simulink model "rightLegController"  (R2017b)
settings: Solver=VariableStepAuto  StartTime=0.0  StopTime=10.0  RelTol=1e-3
libraries: simulink x9, nesl_utility x9
settings Model: Creator=Kalana  LastModifiedBy=Kalana

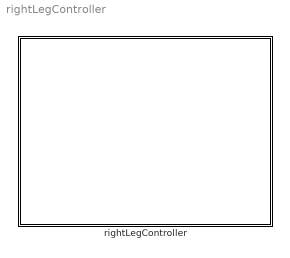
== system rightLegController ==
  "rightLegController " : Subsystem

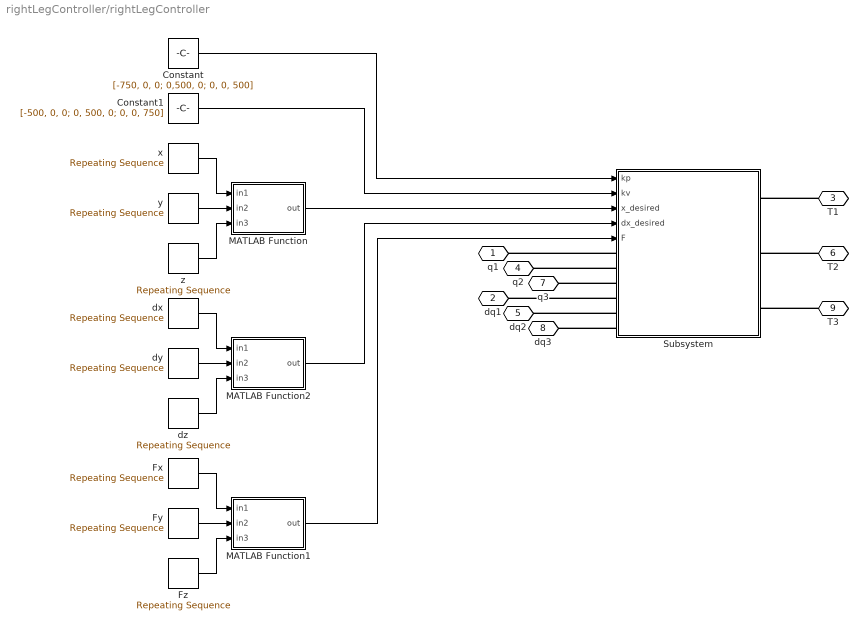
== system rightLegController/rightLegController  ==
  Constant : Constant  Value=[-750, 0, 0; 0,500, 0; 0, 0, 500]  VectorParams1D=off
  Constant1 : Constant  Value=[-500, 0, 0; 0, 500, 0; 0, 0, 750]  VectorParams1D=off
  Fx : simulink/Sources/Repeating Sequence  rep_seq_t=time_force  rep_seq_y=Fx
  Fy : simulink/Sources/Repeating Sequence  rep_seq_t=time_force  rep_seq_y=Fy
  Fz : simulink/Sources/Repeating Sequence  rep_seq_t=time_force  rep_seq_y=Fz
  MATLAB Function : MATLAB Function  TreatAsAtomicUnit=on
  MATLAB Function1 : MATLAB Function  TreatAsAtomicUnit=on
  MATLAB Function2 : MATLAB Function  TreatAsAtomicUnit=on
  Subsystem : Subsystem
  dx : simulink/Sources/Repeating Sequence  rep_seq_t=time_velo  rep_seq_y=Vx
  dy : simulink/Sources/Repeating Sequence  rep_seq_t=time_velo  rep_seq_y=Vy
  dz : simulink/Sources/Repeating Sequence  rep_seq_t=time_velo  rep_seq_y=Vz
  x : simulink/Sources/Repeating Sequence  rep_seq_t=time_pos  rep_seq_y=x
  y : simulink/Sources/Repeating Sequence  rep_seq_t=time_pos  rep_seq_y=y
  z : simulink/Sources/Repeating Sequence  rep_seq_t=time_pos  rep_seq_y=z
  q1 : PMIOPort  Port=1  Side=Left
  dq1 : PMIOPort  Port=2  Side=Left
  T1 : PMIOPort  Port=3  Side=Right
  q2 : PMIOPort  Port=4  Side=Left
  dq2 : PMIOPort  Port=5  Side=Left
  T2 : PMIOPort  Port=6  Side=Right
  q3 : PMIOPort  Port=7  Side=Left
  dq3 : PMIOPort  Port=8  Side=Left
  T3 : PMIOPort  Port=9  Side=Right
  wires:
  y/1 -> MATLAB Function/2(in2)
  x/1 -> MATLAB Function/1(in1)
  dx/1 -> MATLAB Function2/1(in1)
  dy/1 -> MATLAB Function2/2(in2)
  dz/1 -> MATLAB Function2/3(in3)
  z/1 -> MATLAB Function/3(in3)
  Fx/1 -> MATLAB Function1/1(in1)
  Fy/1 -> MATLAB Function1/2(in2)
  Fz/1 -> MATLAB Function1/3(in3)
  MATLAB Function1/1(out) -> Subsystem/5(F)
  MATLAB Function2/1(out) -> Subsystem/4(dx_desired)
  MATLAB Function/1(out) -> Subsystem/3(x_desired)
  Constant/1 -> Subsystem/1(kp)
  Constant1/1 -> Subsystem/2(kv)
  connections:
  Subsystem/LConn4 -- dq1/RConn1
  T3/RConn1 -- Subsystem/RConn3
  T2/RConn1 -- Subsystem/RConn2
  T1/RConn1 -- Subsystem/RConn1
  Subsystem/LConn1 -- q1/RConn1
  Subsystem/LConn2 -- q2/RConn1
  Subsystem/LConn5 -- dq2/RConn1
  Subsystem/LConn3 -- q3/RConn1
  Subsystem/LConn6 -- dq3/RConn1

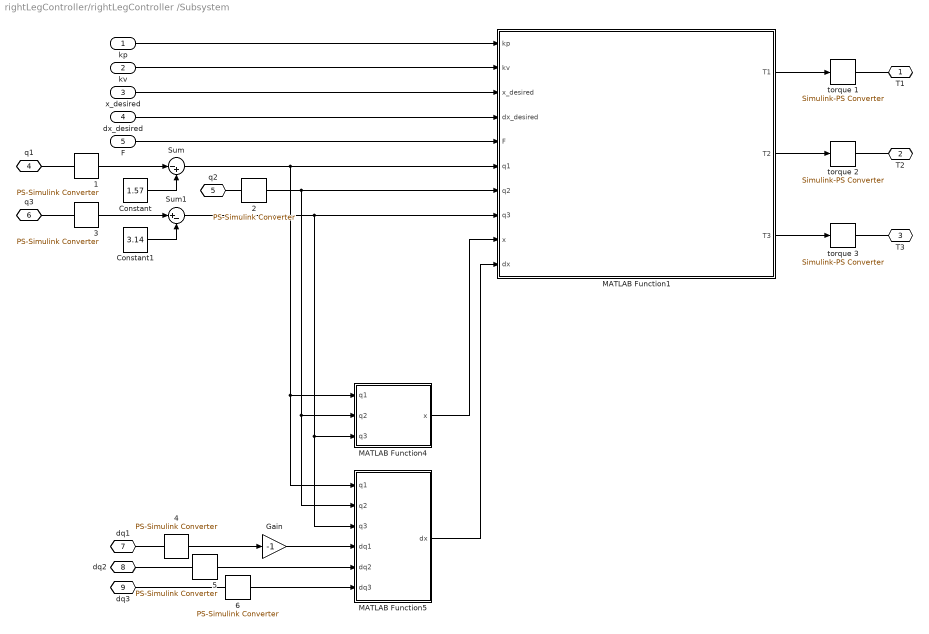
== system rightLegController/rightLegController /Subsystem ==
  kp : Inport
  kv : Inport  Port=2
  x_desired : Inport  Port=3
  dx_desired : Inport  Port=4
  F : Inport  Port=5
  1 : nesl_utility/PS-Simulink Converter  PhysicalDomain=network_engine_domain  SubClassName=ps_output  LeftPortType=input  RightPortType=output  PseudoPeriodic=off  Frequencies=[]  Unit=rad  AffineConversion=off
  2 : nesl_utility/PS-Simulink Converter  PhysicalDomain=network_engine_domain  SubClassName=ps_output  LeftPortType=input  RightPortType=output  PseudoPeriodic=off  Frequencies=[]  Unit=rad  AffineConversion=off
  3 : nesl_utility/PS-Simulink Converter  PhysicalDomain=network_engine_domain  SubClassName=ps_output  LeftPortType=input  RightPortType=output  PseudoPeriodic=off  Frequencies=[]  Unit=rad  AffineConversion=off
  4 : nesl_utility/PS-Simulink Converter  PhysicalDomain=network_engine_domain  SubClassName=ps_output  LeftPortType=input  RightPortType=output  PseudoPeriodic=off  Frequencies=[]  Unit=rad/s  AffineConversion=off
  5 : nesl_utility/PS-Simulink Converter  PhysicalDomain=network_engine_domain  SubClassName=ps_output  LeftPortType=input  RightPortType=output  PseudoPeriodic=off  Frequencies=[]  Unit=rad/s  AffineConversion=off
  6 : nesl_utility/PS-Simulink Converter  PhysicalDomain=network_engine_domain  SubClassName=ps_output  LeftPortType=input  RightPortType=output  PseudoPeriodic=off  Frequencies=[]  Unit=rad/s  AffineConversion=off
  Constant : Constant  Value=1.57
  Constant1 : Constant  Value=3.14
  Gain : Gain  Gain=-1
  MATLAB Function1 : MATLAB Function  TreatAsAtomicUnit=on
  MATLAB Function4 : MATLAB Function  TreatAsAtomicUnit=on
  MATLAB Function5 : MATLAB Function  TreatAsAtomicUnit=on
  Sum : Sum  Inputs=|-+
  Sum1 : Sum  Inputs=|+-
  "torque 1 " : nesl_utility/Simulink-PS Converter  PhysicalDomain=network_engine_domain  SubClassName=ps_input  LeftPortType=input  RightPortType=output  PseudoPeriodic=off  Frequencies=[]  NoiseDistribution=none  NoiseParameters=[]  Unit=N*m  AffineConversion=off  FilteringAndDerivatives=provide  SimscapeFilterOrder=1  InputFilterTimeConstant=0.001  UdotUserProvided=0
  torque 2 : nesl_utility/Simulink-PS Converter  PhysicalDomain=network_engine_domain  SubClassName=ps_input  LeftPortType=input  RightPortType=output  PseudoPeriodic=off  Frequencies=[]  NoiseDistribution=none  NoiseParameters=[]  Unit=N*m  AffineConversion=off  FilteringAndDerivatives=provide  SimscapeFilterOrder=1  InputFilterTimeConstant=0.001  UdotUserProvided=0
  torque 3 : nesl_utility/Simulink-PS Converter  PhysicalDomain=network_engine_domain  SubClassName=ps_input  LeftPortType=input  RightPortType=output  PseudoPeriodic=off  Frequencies=[]  NoiseDistribution=none  NoiseParameters=[]  Unit=N*m  AffineConversion=off  FilteringAndDerivatives=provide  SimscapeFilterOrder=1  InputFilterTimeConstant=0.001  UdotUserProvided=0
  T1 : PMIOPort  Port=1  Side=Right
  T2 : PMIOPort  Port=2  Side=Right
  T3 : PMIOPort  Port=3  Side=Right
  q1 : PMIOPort  Port=4  Side=Left
  q2 : PMIOPort  Port=5  Side=Left
  q3 : PMIOPort  Port=6  Side=Left
  dq1 : PMIOPort  Port=7  Side=Left
  dq2 : PMIOPort  Port=8  Side=Left
  dq3 : PMIOPort  Port=9  Side=Left
  wires:
  3/1 -> Sum1/1
  Constant1/1 -> Sum1/2
  Constant/1 -> Sum/2
  x_desired/1 -> MATLAB Function1/3(x_desired)
  dx_desired/1 -> MATLAB Function1/4(dx_desired)
  MATLAB Function4/1(x) -> MATLAB Function1/9(x)
  MATLAB Function1/3(T3) -> torque 3/1
  6/1 -> MATLAB Function5/6(dq3)
  Sum1/1 -> MATLAB Function5/3(q3), MATLAB Function4/3(q3), MATLAB Function1/8(q3)
  Sum/1 -> MATLAB Function1/6(q1), MATLAB Function5/1(q1), MATLAB Function4/1(q1)
  2/1 -> MATLAB Function5/2(q2), MATLAB Function4/2(q2), MATLAB Function1/7(q2)
  5/1 -> MATLAB Function5/5(dq2)
  MATLAB Function1/1(T1) -> "torque 1 "/1
  MATLAB Function5/1(dx) -> MATLAB Function1/10(dx)
  MATLAB Function1/2(T2) -> torque 2/1
  F/1 -> MATLAB Function1/5(F)
  kp/1 -> MATLAB Function1/1(kp)
  kv/1 -> MATLAB Function1/2(kv)
  1/1 -> Sum/1
  4/1 -> Gain/1
  Gain/1 -> MATLAB Function5/4(dq1)
  connections:
  4/LConn1 -- dq1/RConn1
  2/LConn1 -- q2/RConn1
  "torque 1 "/RConn1 -- T1/RConn1
  torque 2/RConn1 -- T2/RConn1
  1/LConn1 -- q1/RConn1
  torque 3/RConn1 -- T3/RConn1
  3/LConn1 -- q3/RConn1
  6/LConn1 -- dq3/RConn1
  5/LConn1 -- dq2/RConn1

== matlab function rightLegController/rightLegController /Subsystem/MATLAB Function1 ==
  data: kp input; kv input; x_desired input; dx_desired input; F input; T1 output; q1 input; q2 input; q3 input; x input; dx input; T2 output; T3 output
function [T1, T2, T3] = rightLegControl(kp, kv, x_desired, dx_desired, F, q1, q2, q3, x, dx)

g = [0     ;
     -9.8;
     0     ];

Mass_1 = [1.13997,  0,        0;
          0,        1.13997,  0;
          0,        0,        1.13997];

Iner_1 = [ 4695654.71e-09,      -3171848.05e-09,     212.52e-09;
           -3171848.05e-09,     4943364.65e-09,      -363.95e-09;
           212.52e-09,          -363.95e-09,         8566375.52e-09];

      
Mass_2 = [1.13649,  0,        0;
          0,        1.13649,  0;
          0,        0,        1.13649];

Iner_2 = [2554474.68e-09,      -231.05e-09,         -2855264.81e-09;
          -231.05e-09,         12519194.41e-09,     8.54e-09;
          -2855264.81e-09,     8.54e-09,            10576743.61e-09];

      
Mass_3 = [0.63820,  0,        0;
          0,        0.63820,  0;
          0,        0,        0.63280];
  
Iner_3 = [728680.81e-09,      -172.39e-09,        158.48e-09;
          -172.39e-09,        2618699.35e-09,     -3.33e-09;
          158.48e-09,         -3.33e-09,          2391085.66e-09];

      
Jv1 = [0.05737*cos(q1)-0.05549*sin(q1),    0, 0;
       0.05737*sin(q1)+0.05549*cos(q1),    0, 0;
       0,                                  0, 0];

Jw1 = [0, 0, 0;
       0, 0, 0;
       1, 0, 0];

   
Jv2 = [-0.09947*sin(q1)*cos(q2)+0.08747*cos(q1)-0.1225*sin(q1),  -0.09947*cos(q1)*sin(q2),      0;
       0.09947*cos(q1)*cos(q2)+0.08747*sin(q1)+0.1225*cos(q1),   -0.09947*sin(q1)*sin(q2),      0; 
       0,                                                        -0.09947*cos(q2),              0]; 
      
Jw2 = [0, -1, 0; 
       0,  0, 0; 
       1,  0, 0];
 
   
Jv3 = [-0.02559*sin(q1)*cos(q2-q3)-0.2*sin(q1)*cos(q2)-0.1225*sin(q1)+0.0525*cos(q1),  -0.02559*cos(q1)*sin(q2-q3)-0.2*cos(q1)*sin(q2),  0.02559*cos(q1)*sin(q2-q3);
       0.02559*cos(q1)*cos(q2-q3)+0.2*cos(q1)*cos(q2)+0.1225*cos(q1)+0.0525*sin(q1),   -0.02559*sin(q1)*sin(q2-q3)-0.2*sin(q1)*sin(q2),  0.02559*sin(q1)*sin(q2-q3);
       0,                                                                              -0.02559*cos(q2-q3)-0.2*cos(q2),                  0.02559*cos(q2-q3)       ];
      
Jw3 = [0, -1, 1;
       0,  0, 0;
       1,  0, 0];

   
JvEE = [-0.245*sin(q1)*cos(q2-q3)-0.2*sin(q1)*cos(q2)-0.1225*sin(q1)+0.0525*cos(q1),  -0.245*cos(q1)*sin(q2-q3)-0.2*cos(q1)*sin(q2),  0.245*cos(q1)*sin(q2-q3);
        0.245*cos(q1)*cos(q2-q3)+0.2*cos(q1)*cos(q2)+0.1225*cos(q1)+0.0525*sin(q1),   -0.245*sin(q1)*sin(q2-q3)-0.2*sin(q1)*sin(q2),  0.245*sin(q1)*sin(q2-q3);
        0,                                                                            -0.245*cos(q2-q3)-0.2*cos(q2),                  0.245*cos(q2-q3)       ];
   

Mass_q = Jv1'*Mass_1*Jv1 + Jw1'*Iner_1*Jw1 + Jv2'*Mass_2*Jv2 + Jw2'*Iner_2*Jw2 + Jv3'*Mass_3*Jv3 + Jw3'*Iner_3*Jw3;

Mass_x = JvEE'*pinv(JvEE*(inv(Mass_q))*JvEE');

Grav = Jv1'*Mass_1*g + Jv2'*Mass_2*g + Jv3'*Mass_3*g;

Force = JvEE'*F;

torque = Mass_x*((kp*(x_desired - x)) + (kv*(dx_desired - dx))) + Grav;

T1 = torque(1);
T2 = torque(2);
T3 = torque(3);

== matlab function rightLegController/rightLegController /MATLAB Function ==
  data: in1 input; out output; in2 input; in3 input
function out = matrix(in1, in2, in3)
out = [in1; in2; in3];

== matlab function rightLegController/rightLegController /MATLAB Function1 ==
  data: in1 input; out output; in2 input; in3 input
function out = matrix(in1, in2, in3)
out = [in1; in2; in3];

== matlab function rightLegController/rightLegController /MATLAB Function2 ==
  data: in1 input; out output; in2 input; in3 input
function out = matrix(in1, in2, in3)
out = [in1; in2; in3];

== matlab function rightLegController/rightLegController /Subsystem/MATLAB Function4 ==
  data: q1 input; x output; q2 input; q3 input
function x = Kinematics(q1, q2, q3)

leg = [0.245;
       0;
       0;
       1];
   
Trans0_3 = [cos(q1)*cos(q2-q3),    cos(q1)*sin(q2-q3),    sin(q1),       0.2*cos(q1)*cos(q2)+0.1225*cos(q1)+0.0525*sin(q1);
            sin(q1)*cos(q2-q3),    sin(q1)*sin(q2-q3),    -cos(q1),      0.2*sin(q1)*cos(q2)+0.1225*sin(q1)-0.0525*cos(q1);
            -sin(q2-q3),           cos(q2-q3),            0,             -0.2*sin(q2);
            0,                      0,                    0,              1];
        
x_temp = Trans0_3*leg;

x = x_temp(1:3);

== matlab function rightLegController/rightLegController /Subsystem/MATLAB Function5 ==
  data: q1 input; dx output; q2 input; q3 input; dq1 input; dq2 input; dq3 input
function dx = Jacobian(q1, q2, q3, dq1, dq2, dq3)

dq = [ dq1;
       dq2;
       dq3];

JvEE = [-0.245*sin(q1)*cos(q2-q3)-0.2*sin(q1)*cos(q2)-0.1225*sin(q1)+0.0525*cos(q1),  -0.245*cos(q1)*sin(q2-q3)-0.2*cos(q1)*sin(q2),  0.245*cos(q1)*sin(q2-q3);
        0.245*cos(q1)*cos(q2-q3)+0.2*cos(q1)*cos(q2)+0.1225*cos(q1)+0.0525*sin(q1),   -0.245*sin(q1)*sin(q2-q3)-0.2*sin(q1)*sin(q2),  0.245*sin(q1)*sin(q2-q3);
        0,                                                                            -0.245*cos(q2-q3)-0.2*cos(q2),                  0.245*cos(q2-q3)       ];
   
dx = JvEE*dq;
